simulink model "Lab07es01_schema"  (R2021a)
settings: Solver=VariableStepAuto  StartTime=0.0  StopTime=10  RelTol=1e-3
values from neighbouring files (symbols this model uses):
  Kr = 1    [L_11_05_21_reti_anticipatrici.m]    (also in L_11_05_21_reti_anticipatrici_2.m; L_12_05_21_Esercizio_progetto_di_un_controllore.m; L_12_05_21_effetti_sul_comando.m; L_12_05_21_reti_integro-derivative.m)
libraries: cstblocks x2, simulink x1
settings Model: Creator=armandofornasier  LastModifiedBy=armandofornasier

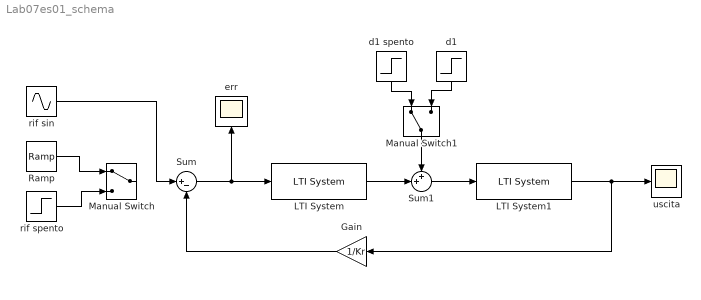
== system Lab07es01_schema ==
  Gain : Gain  Gain=1/Kr
  LTI System : cstblocks/LTI System  sys=C  IC=[]
  LTI System1 : cstblocks/LTI System  sys=F  IC=[]
  Manual Switch : ManualSwitch
  Manual Switch1 : ManualSwitch
  Ramp : simulink/Sources/Ramp  slope=1  start=0  InitialOutput=0
  Sum : Sum  Inputs=|+-
  Sum1 : Sum  Inputs=++|
  d1 : Step  Time=0  SampleTime=0
  d1 spento : Step  Time=0  After=0  SampleTime=0
  err : Scope
  rif sin : Sin  Frequency=100  SampleTime=0
  rif spento : Step  Time=0  After=0  SampleTime=0
  uscita : Scope
  wires:
  LTI System/1 -> Sum1/2
  Sum1/1 -> LTI System1/1
  LTI System1/1 -> Gain/1, uscita/1
  Sum/1 -> err/1, LTI System/1
  Ramp/1 -> Manual Switch/1
  Gain/1 -> Sum/2
  rif spento/1 -> Manual Switch/2
  Manual Switch1/1 -> Sum1/1
  d1 spento/1 -> Manual Switch1/1
  d1/1 -> Manual Switch1/2
  rif sin/1 -> Sum/1
